simulink library "arc"  (R2023b)
settings: Solver=VariableStepAuto  StartTime=0.0  StopTime=10.0  RelTol=1e-3
values from neighbouring files (symbols this model uses):
  AF = 0.90    (= 0.9)    [FC_scenario_inputData.m]    (also in inputData.m = 70)
  eta2 = 0.95    [FC_scenario_inputData.m]    (also in inputData.m)
  f51 = 0.33    [FC_scenario_inputData.m]    (also in inputData.m)
  f53 = 0.33    [FC_scenario_inputData.m]    (also in inputData.m)
  f54 = 1 - f51 - f53 - f56    (= 0.3399)    [FC_scenario_inputData.m]    (also in inputData.m)
  f56 = 1e-4    (= 0.0001)    [FC_scenario_inputData.m]    (also in inputData.m)
  f96 = 0.1    [FC_scenario_inputData.m]    (also in inputData.m)
  f_dir = 0.7    [FC_scenario_inputData.m]    (also in inputData.m = 0.3)
  f_permanent_trap = f_permanent_trap_array(i)    [parametric_analysis_trapping.m]
  fp3 = 1e-4    (= 0.0001)    [FC_scenario_inputData.m]    (also in inputData.m; parametric_analysis_f_p_trap.m = f_p(i))
  fp4 = 1e-4    (= 0.0001)    [FC_scenario_inputData.m]    (also in inputData.m; parametric_analysis_f_p_trap.m = f_p(i))
  I_s_0 = 1.85    [fuelCycleSimulator.m]    (also in parametric_analysis_f_p_trap.m = 0.8; utilities.m = I_s_0 - abs(margin) + inventory_accuracy)
  lambda = 1.73e-9    (= 1.73e-09)    [FC_scenario_inputData.m]    (also in inputData.m)
  M_structural = V_structural * rho_structural/1e3    (= 21350)    [inputData_trapping.m]
  M_tungsten = V_tungsten * rho_tungsten/1e3    (= 6755)    [inputData_trapping.m]
  m_u = 1.6e-27    [inputData_trapping.m]
  N_dot = 9.3e-7    (= 9.3e-07)    [FC_scenario_inputData.m]    (also in inputData.m)
  n_solute_tungsten = 6    [inputData_trapping.m]
  n_structural = (rho_structural*1e6) / PM_structural * N_a    (= 7.36894684052e+28)    [inputData_trapping.m]
  n_trap = n_trap_array(j)    [parametric_analysis_trapping.m]
  n_trap_structural = n_trap_vcrti    (= 0.0001)    [inputData_trapping.m]    (also in parametric_analysis_trapping.m = n_trap_array(j))
  n_tungsten = (rho_tungsten*1e6) / PM_tungsten * N_a    (= 6.32342763874e+28)    [inputData_trapping.m]
  PM_structural = PM_vcrti    (= 49.85)    [inputData_trapping.m]
  PM_tritium = 3    [inputData_trapping.m]
  PM_tungsten = 183.8    [inputData_trapping.m]
  T1 = 1/((1 + epsi)/tau1 + lambda)    [FC_scenario_inputData.m]    (also in inputData.m)
  T12 = 1/((1 + epsi)/tau12 + lambda)    [FC_scenario_inputData.m]    (also in inputData.m)
  T2 = 1/((1 + epsi)/tau2 + lambda)    [FC_scenario_inputData.m]    (also in inputData.m)
  T3 = 1/((1 + 0)/tau3 + lambda)    [FC_scenario_inputData.m]    (also in inputData.m)
  T4 = 1/((1 + 0)/tau4 + lambda)    [FC_scenario_inputData.m]    (also in inputData.m)
  T5 = 1/((1 + epsi)/tau5 + lambda)    [FC_scenario_inputData.m]    (also in inputData.m)
  T6 = 1/((1 + epsi)/tau6 + lambda)    [FC_scenario_inputData.m]    (also in inputData.m)
  T7 = 1/((1 + epsi)/tau7 + lambda)    [FC_scenario_inputData.m]    (also in inputData.m)
  T9 = 1/((1 + epsi)/tau9 + lambda)    [FC_scenario_inputData.m]    (also in inputData.m)
  T_replacement = 1.7*8760*3600    (= 53611200)    [inputData.m]
  tau1 = 1.25*3600    (= 4500)    [FC_scenario_inputData.m]    (also in inputData.m)
  tau12 = 100    [FC_scenario_inputData.m]    (also in inputData.m)
  tau2 = 1*24*3600    (= 86400)    [FC_scenario_inputData.m]    (also in inputData.m)
  tau3 = 1000    [FC_scenario_inputData.m]    (also in inputData.m)
  tau4 = 1000    [FC_scenario_inputData.m]    (also in inputData.m)
  tau5 = 1000    [FC_scenario_inputData.m]    (also in inputData.m)
  tau6 = 3600    [FC_scenario_inputData.m]    (also in inputData.m)
  tau7 = 600    [FC_scenario_inputData.m]    (also in inputData.m)
  tau8 = 0.1*3600    (= 360)    [FC_scenario_inputData.m]    (also in inputData.m = 3600)
  tau9 = 0.9*3600    (= 3240)    [FC_scenario_inputData.m]    (also in inputData.m = 10800)
  tau_detrap_structural = 1 / nu_detrap_structural* relaxation_coefficient    [inputData_trapping.m]
  tau_detrap_tungsten = 1 ./ nu_detrap* relaxation_coefficient    [inputData_trapping.m]
  tau_trap_structural = 1/nu_trap_structural * relaxation_coefficient    [inputData_trapping.m]
  tau_trap_tungsten = 1/nu_trap * relaxation_coefficient    [inputData_trapping.m]
  TBE = 0.02    [FC_scenario_inputData.m]    (also in inputData.m; parametric_analysis_f_p_trap.m = TBE_array(j); parametric_analysis_trapping.m)
  TBR = 1.096    [fuelCycleSimulator.m]    (also in parametric_analysis_f_p_trap.m = 1.048; parametric_analysis_trapping.m = 1.06; utilities.m = TBR_start)
  V_structural = 3.5e6    (= 3500000)    [inputData_trapping.m]
undefined symbols (not defined in the file or in its folder): f_permanent_trap_structural, n_solute, tau_detrap, tau_permanent, tau_permanent_structural
libraries: $bdroot x4
settings Model: Creator=smesc  LastModifiedBy=meschini
settings OptimizationCC: ReuseModelBlockBuffer=off
settings ModelReferenceCC: EnableRefExpFcnMdlSchedulingChecks=on

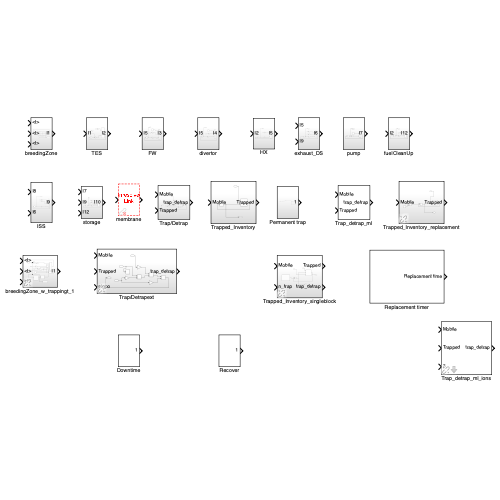
[thumbnail: Simulink's stored preview of the top-level diagram]
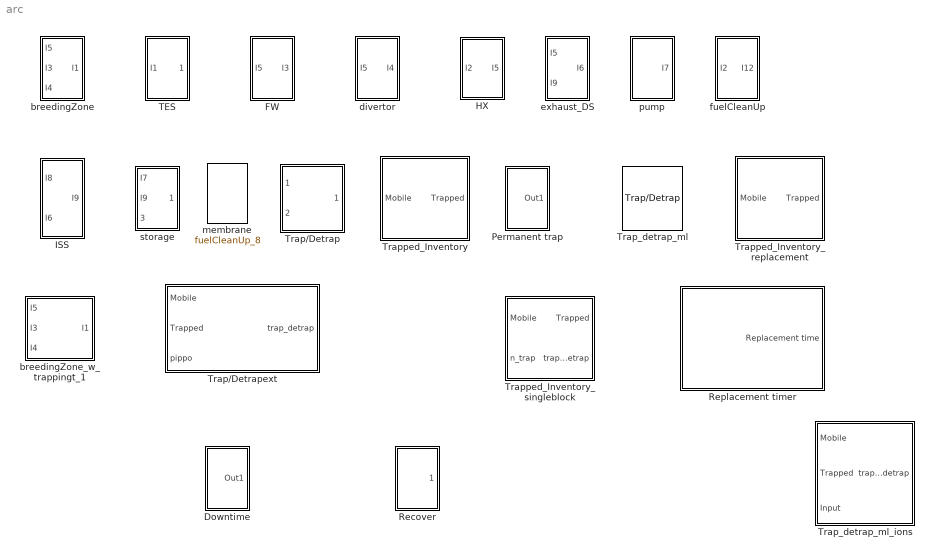
== system arc ==
  Downtime : Subsystem  mask{T_shutdown=0, T_restart=0}
      mask prompts: T_shutdown "Time at which reactor is shutdown"; T_restart "Time at which reactor restarts"
  FW : Subsystem
      settings: LibrarySourceBlock=arc/FW_3
  HX : Subsystem
  ISS : Subsystem
      settings: LibrarySourceBlock=arc/ISS_9
  Permanent trap : Subsystem
  Recover : Subsystem  mask{T_recover_start=0, T_recover_stop=0}
      mask prompts: T_recover_start "Start recover phase"; T_recover_stop "Stop recover phase"
  Replacement timer : Subsystem  mask{T_replacement=T_replacement}
      mask prompts: T_replacement "Replacement time"
  TES : Subsystem
      settings: LibrarySourceBlock=arc/TES_2
  Trap/Detrap : Subsystem
  Trap/Detrapext : Subsystem  AncestorBlock=arc/Trap//Detrap
  Trap_detrap_ml : $bdroot/Trap//Detrap  mask{n_trap=0, tau_trap=0, tau_detrap=0, n_solute=0, PM_host=0, PM_tritium=0, M_host=0}
      mask prompts: n_trap "Trap density"; tau_trap "Tau trap"; tau_detrap "Tau detrap"; PM_host "PM host"; PM_tritium "PM T"
  Trap_detrap_ml_ions : Subsystem  AncestorBlock=arc/Trapped_Inventory_singleblock/Trap_detrap_ml2  mask{tau_trap=tau_trap_tungsten, tau_detrap=tau_detrap_tungsten(1), n_solute=n_solute_tungsten, PM_host=PM_tungsten, PM_tritium=PM_tritium, M_host=M_tungsten, fp=0}
      mask prompts: tau_trap "Tau trap"; tau_detrap "Tau detrap"; PM_host "PM host"; PM_tritium "PM T"; fp "Ions impinging to walls"
  Trapped_Inventory : Subsystem
  Trapped_Inventory_replacement : Subsystem  AncestorBlock=arc/Trapped_Inventory
  Trapped_Inventory_singleblock : Subsystem  AncestorBlock=arc/Trapped_Inventory
  breedingZone : Subsystem
      settings: LibrarySourceBlock=arc/breedingZone_1
  breedingZone_w_trappingt_1 : Subsystem  AncestorBlock=arc/breedingZone_1
      settings: LibrarySourceBlock=arc/breedingZone_1
  divertor : Subsystem
      settings: LibrarySourceBlock=arc/divertor_4
  exhaust_DS : Subsystem
  fuelCleanUp : Subsystem
      settings: LibrarySourceBlock=arc/fuelCleanUp_8
  membrane : $bdroot/fuelCleanUp_8  SystemSampleTime=-1  SSRTWFcnClass=[]  VariantActivationTime=update diagram  Latency=0  AutoFrameSizeCalculation=off
      settings: LibrarySourceBlock=arc/fuelCleanUp_8
  pump : Subsystem
      settings: LibrarySourceBlock=arc/pump_7
  storage : Subsystem
      settings: LibrarySourceBlock=arc/storage_10

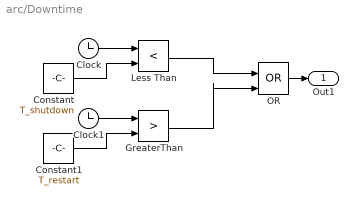
== system arc/Downtime ==
  Clock : Clock
  Clock1 : Clock
  Constant : Constant  Value=T_shutdown
  Constant1 : Constant  Value=T_restart
  GreaterThan : RelationalOperator  Operator=>  OutDataTypeStr=boolean  RndMeth=Simplest  InputSameDT=off
  Less Than : RelationalOperator  Operator=<  OutDataTypeStr=boolean  RndMeth=Simplest  InputSameDT=off
  OR : Logic  Operator=OR  IconShape=distinctive  AllPortsSameDT=off  OutDataTypeStr=boolean
  Out1 : Outport
  wires:
  OR/1 -> Out1/1
  Constant/1 -> Less Than/2
  GreaterThan/1 -> OR/2
  Clock/1 -> Less Than/1
  Clock1/1 -> GreaterThan/1
  Constant1/1 -> GreaterThan/2
  Less Than/1 -> OR/1

== system arc/FW ==
  I5 : Inport
  Add : Sum  Inputs=++-
  Gain : Gain  Gain=f53/tau5
  Gain2 : Gain  Gain=1/T3
  Integrator : Integrator
  Pulse Generator : DiscretePulseGenerator  PulseType=Time based  Amplitude=fp3*N_dot/TBE  Period=1800  PulseWidth=AF
  I3 : Outport
  wires:
  I5/1 -> Gain/1
  Gain/1 -> Add/2
  Add/1 -> Integrator/1  "I_dot"
  Integrator/1 -> Gain2/1, I3/1  "I"
  Pulse Generator/1 -> Add/1
  Gain2/1 -> Add/3

== system arc/HX ==
  I2 : Inport
  Add : Sum  Inputs=+-
  Gain : Gain  Gain=(1-eta2)/tau2
  Gain3 : Gain  Gain=1/T5
  Integrator : Integrator
  I5 : Outport
  wires:
  I2/1 -> Gain/1
  Gain3/1 -> Add/2
  Gain/1 -> Add/1
  Add/1 -> Integrator/1  "I_dot"
  Integrator/1 -> I5/1, Gain3/1  "I"

== system arc/ISS ==
  I8 : Inport
  I6 : Inport  Port=2
  Add : Sum  Inputs=++-
  Gain : Gain  Gain=1/tau8
  Gain1 : Gain  Gain=1/tau6
  Gain4 : Gain  Gain=1/T9
  Integrator : Integrator
  I9 : Outport
  wires:
  Gain4/1 -> Add/3
  Gain/1 -> Add/1
  Integrator/1 -> I9/1, Gain4/1  "I"
  Add/1 -> Integrator/1  "I_dot"
  I6/1 -> Gain1/1
  Gain1/1 -> Add/2
  I8/1 -> Gain/1

== system arc/Permanent trap ==
  Clock : Clock
  Exp : Math
  Gain1 : Gain  Gain=-1/tau_permanent
  Gain3 : Gain  Gain=f_permanent_trap*n_trap*n_tungsten*3*m_u*1/tau_permanent
  Scope : Scope
  Out1 : Outport
  wires:
  Exp/1 -> Gain3/1
  Gain3/1 -> Scope/1, Out1/1
  Clock/1 -> Gain1/1
  Gain1/1 -> Exp/1

== system arc/Recover ==
  AND : Logic  IconShape=distinctive  AllPortsSameDT=off  OutDataTypeStr=boolean
  Clock : Clock
  Clock1 : Clock
  Constant : Constant  Value=T_recover_stop
  Constant1 : Constant  Value=T_recover_start
  GreaterThan : RelationalOperator  Operator=>  OutDataTypeStr=boolean  RndMeth=Simplest  InputSameDT=off
  Less Than : RelationalOperator  Operator=<  OutDataTypeStr=boolean  RndMeth=Simplest  InputSameDT=off
  Output : Outport
  wires:
  GreaterThan/1 -> AND/2
  Clock/1 -> Less Than/1
  AND/1 -> Output/1
  Clock1/1 -> GreaterThan/1
  Constant/1 -> Less Than/2
  Constant1/1 -> GreaterThan/2
  Less Than/1 -> AND/1

== system arc/Replacement timer ==
  Clock : Clock
  Constant1 : Constant  Value=T_replacement
  Rem : Math  Operator=mod
  Replacement time : Outport
  wires:
  Clock/1 -> Rem/1
  Constant1/1 -> Rem/2
  Rem/1 -> Replacement time/1

== system arc/TES ==
  I1 : Inport
  Add : Sum  Inputs=+-
  Gain : Gain  Gain=1/T2
  Gain1 : Gain  Gain=1/tau1
  Integrator : Integrator
  Output : Outport
  wires:
  Add/1 -> Integrator/1  "I_dot"
  Integrator/1 -> Output/1, Gain/1  "I2"
  Gain1/1 -> Add/1
  I1/1 -> Gain1/1
  Gain/1 -> Add/2

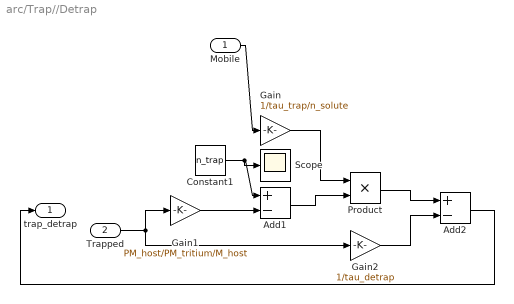
== system arc/Trap//Detrap ==
  Mobile : Inport
  Trapped : Inport  Port=2
  Add1 : Sum  Inputs=+-
  Add2 : Sum  Inputs=+-
  Constant1 : Constant  Value=n_trap
  Gain : Gain  Gain=1/tau_trap/n_solute
  Gain1 : Gain  Gain=PM_host/PM_tritium/M_host
  Gain2 : Gain  Gain=1/tau_detrap
  Product : Product
  Scope : Scope
  trap_detrap : Outport
  wires:
  Product/1 -> Add2/1
  Add2/1 -> trap_detrap/1
  Mobile/1 -> Gain/1
  Gain/1 -> Product/1
  Constant1/1 -> Scope/1, Add1/1
  Gain2/1 -> Add2/2
  Add1/1 -> Product/2
  Gain1/1 -> Add1/2
  Trapped/1 -> Gain2/1, Gain1/1

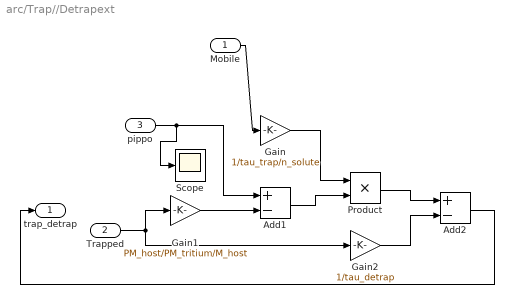
== system arc/Trap//Detrapext ==
  Mobile : Inport
  Trapped : Inport  Port=2
  pippo : Inport  Port=3
  Add1 : Sum  Inputs=+-
  Add2 : Sum  Inputs=+-
  Gain : Gain  Gain=1/tau_trap/n_solute
  Gain1 : Gain  Gain=PM_host/PM_tritium/M_host
  Gain2 : Gain  Gain=1/tau_detrap
  Product : Product
  Scope : Scope
  trap_detrap : Outport
  wires:
  Product/1 -> Add2/1
  Add2/1 -> trap_detrap/1
  Mobile/1 -> Gain/1
  Gain/1 -> Product/1
  pippo/1 -> Scope/1, Add1/1
  Gain2/1 -> Add2/2
  Add1/1 -> Product/2
  Gain1/1 -> Add1/2
  Trapped/1 -> Gain2/1, Gain1/1

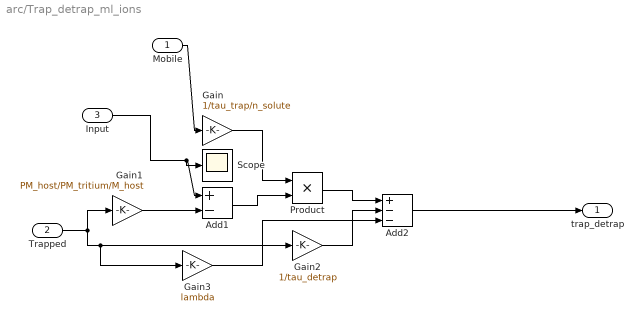
== system arc/Trap_detrap_ml_ions ==
  Mobile : Inport
  Trapped : Inport  Port=2
  Input : Inport  Port=3
  Add1 : Sum  Inputs=+-
  Add2 : Sum  Inputs=+--
  Gain : Gain  Gain=1/tau_trap/n_solute
  Gain1 : Gain  Gain=PM_host/PM_tritium/M_host
  Gain2 : Gain  Gain=1/tau_detrap
  Gain3 : Gain  Gain=lambda
  Product : Product
  Scope : Scope
  trap_detrap : Outport
  wires:
  Trapped/1 -> Gain1/1, Gain2/1, Gain3/1
  Gain1/1 -> Add1/2
  Add1/1 -> Product/2
  Input/1 -> Add1/1, Scope/1
  Gain/1 -> Product/1
  Mobile/1 -> Gain/1
  Add2/1 -> trap_detrap/1
  Product/1 -> Add2/1
  Gain2/1 -> Add2/2
  Gain3/1 -> Add2/3

== system arc/Trapped_Inventory ==
  Mobile : Inport
  Integrator1 : Integrator
  Trap/Detrap : Subsystem
  Trapped : Outport
  wires:
  Integrator1/1 -> Trapped/1, Trap/Detrap/2(In2)
  Mobile/1 -> Trap/Detrap/1(In1)
  Trap/Detrap/1(Out1) -> Integrator1/1

== system arc/Trapped_Inventory_replacement ==
  Mobile : Inport
  Clock : Clock
  Constant1 : Constant  Value=T_replacement
  Integrator1 : Integrator  ExternalReset=falling
  Rem : Math  Operator=mod
  Trap_detrap_ml : $bdroot/Trap_detrap_ml  n_trap=n_trap_structural  tau_trap=tau_trap_structural  tau_detrap=tau_detrap_structural  n_solute=n_solute  PM_host=PM_structural  PM_tritium=PM_tritium  M_host=M_structural
  Trapped : Outport
  wires:
  Mobile/1 -> Trap_detrap_ml/1
  Integrator1/1 -> Trap_detrap_ml/2, Trapped/1
  Clock/1 -> Rem/1
  Rem/1 -> Integrator1/2
  Constant1/1 -> Rem/2
  Trap_detrap_ml/1 -> Integrator1/1

== system arc/Trapped_Inventory_singleblock ==
  Mobile : Inport
  n_trap : Inport  Port=2
  Integrator1 : Integrator  ExternalReset=falling
  Replacement timer : $bdroot/Replacement timer  T_replacement=T_replacement
  Trap_detrap_ml2 : Subsystem  AncestorBlock=arc/Trap_detrap_ml  mask{tau_trap=tau_trap_structural, tau_detrap=tau_detrap_tungsten(3), n_solute=n_solute, PM_host=PM_structural, PM_tritium=PM_tritium, M_host=M_structural}
      mask prompts: tau_trap "Tau trap"; tau_detrap "Tau detrap"; PM_host "PM host"; PM_tritium "PM T"
  Trapped : Outport
  trap_detrap : Outport  Port=2
  wires:
  Integrator1/1 -> Trap_detrap_ml2/2(Trapped), Trapped/1
  Mobile/1 -> Trap_detrap_ml2/1(Mobile)
  Trap_detrap_ml2/1(trap_detrap) -> trap_detrap/1, Integrator1/1
  n_trap/1 -> Trap_detrap_ml2/3(Input)
  Replacement timer/1 -> Integrator1/2

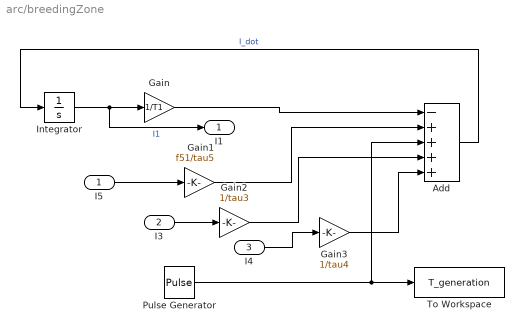
== system arc/breedingZone ==
  I5 : Inport
  I3 : Inport  Port=2
  I4 : Inport  Port=3
  Add : Sum  Inputs=-++++
  Gain : Gain  Gain=1/T1
  Gain1 : Gain  Gain=f51/tau5
  Gain2 : Gain  Gain=1/tau3
  Gain3 : Gain  Gain=1/tau4
  Integrator : Integrator
  Pulse Generator : DiscretePulseGenerator  PulseType=Time based  Amplitude=N_dot * TBR  Period=1800  PulseWidth=AF
  To Workspace : ToWorkspace  VariableName=T_generation  SaveFormat=Timeseries  SampleTime=-1
  I1 : Outport
  wires:
  Gain3/1 -> Add/5
  I4/1 -> Gain3/1
  Gain2/1 -> Add/4
  I3/1 -> Gain2/1
  Pulse Generator/1 -> To Workspace/1, Add/3
  I5/1 -> Gain1/1
  Gain/1 -> Add/1
  Integrator/1 -> I1/1, Gain/1  "I1"
  Gain1/1 -> Add/2
  Add/1 -> Integrator/1  "I_dot"

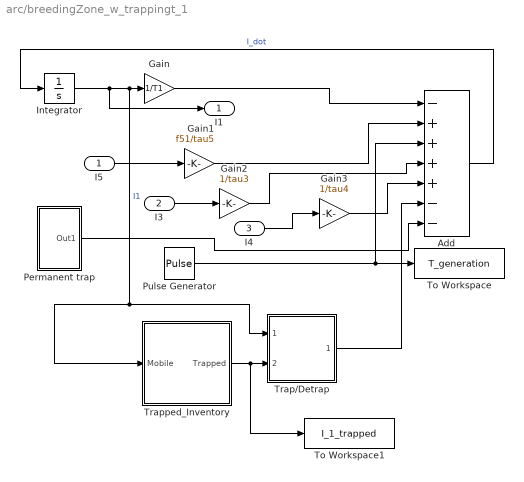
== system arc/breedingZone_w_trappingt_1 ==
  I5 : Inport
  I3 : Inport  Port=2
  I4 : Inport  Port=3
  Add : Sum  Inputs=-++++--
  Gain : Gain  Gain=1/T1
  Gain1 : Gain  Gain=f51/tau5
  Gain2 : Gain  Gain=1/tau3
  Gain3 : Gain  Gain=1/tau4
  Integrator : Integrator
  Permanent trap : Subsystem
  Pulse Generator : DiscretePulseGenerator  PulseType=Time based  Amplitude=N_dot * TBR  Period=1800  PulseWidth=AF
  To Workspace : ToWorkspace  VariableName=T_generation  SaveFormat=Timeseries  SampleTime=-1
  To Workspace1 : ToWorkspace  VariableName=I_1_trapped  SampleTime=-1
  Trap/Detrap : Subsystem  AncestorBlock=arc/Trap//Detrap
  Trapped_Inventory : Subsystem  AncestorBlock=arc/Trapped_Inventory
  I1 : Outport
  wires:
  Add/1 -> Integrator/1  "I_dot"
  Gain1/1 -> Add/2
  Integrator/1 -> Trapped_Inventory/1(Mobile), Trap/Detrap/1(Mobile), Gain/1, I1/1  "I1"
  Gain/1 -> Add/1
  I5/1 -> Gain1/1
  Pulse Generator/1 -> Add/3, To Workspace/1
  I3/1 -> Gain2/1
  Gain2/1 -> Add/4
  I4/1 -> Gain3/1
  Gain3/1 -> Add/5
  Trapped_Inventory/1(Trapped) -> To Workspace1/1, Trap/Detrap/2(Trapped)
  Trap/Detrap/1(trap_detrap) -> Add/6
  Permanent trap/1(Out1) -> Add/7

== system arc/divertor ==
  I5 : Inport
  Add : Sum  Inputs=++-
  Gain : Gain  Gain=f54/tau5
  Gain2 : Gain  Gain=1/T4
  Integrator : Integrator
  Pulse Generator : DiscretePulseGenerator  PulseType=Time based  Amplitude=fp4*N_dot/TBE  Period=1800  PulseWidth=AF
  I4 : Outport
  wires:
  I5/1 -> Gain/1
  Gain2/1 -> Add/3
  Add/1 -> Integrator/1  "I_dot"
  Integrator/1 -> I4/1, Gain2/1  "I"
  Gain/1 -> Add/2
  Pulse Generator/1 -> Add/1

== system arc/exhaust_DS ==
  I5 : Inport
  I9 : Inport  Port=2
  Add : Sum  Inputs=++-
  Gain : Gain  Gain=f56/tau5
  Gain1 : Gain  Gain=f96/tau9
  Gain2 : Gain  Gain=1/T6
  Integrator : Integrator
  I6 : Outport
  wires:
  Gain/1 -> Add/1
  I5/1 -> Gain/1
  Gain1/1 -> Add/2
  Add/1 -> Integrator/1  "I_dot"
  Gain2/1 -> Add/3
  Integrator/1 -> I6/1, Gain2/1  "I"
  I9/1 -> Gain1/1

== system arc/fuelCleanUp ==
  I2 : Inport
  Add : Sum  Inputs=+-
  Gain : Gain  Gain=eta2/tau2
  Gain1 : Gain  Gain=1/T12
  Integrator : Integrator
  I12 : Outport
  wires:
  Gain/1 -> Add/1
  Integrator/1 -> I12/1, Gain1/1  "I"
  Add/1 -> Integrator/1  "I_dot"
  Gain1/1 -> Add/2
  I2/1 -> Gain/1

== system arc/pump ==
  Add : Sum  Inputs=+-
  Gain : Gain  Gain=1/T7
  Integrator : Integrator
  Pulse Generator : DiscretePulseGenerator  PulseType=Time based  Amplitude=(1-TBE-fp3-fp4)*N_dot/TBE  Period=1800  PulseWidth=AF
  I7 : Outport
  wires:
  Add/1 -> Integrator/1  "I_dot"
  Pulse Generator/1 -> Add/1
  Integrator/1 -> I7/1, Gain/1  "I7"
  Gain/1 -> Add/2

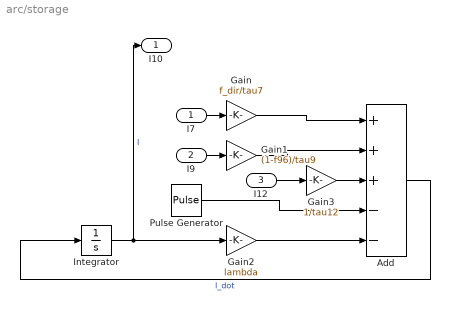
== system arc/storage ==
  I7 : Inport
  I9 : Inport  Port=2
  I12 : Inport  Port=3
  Add : Sum  Inputs=+++--
  Gain : Gain  Gain=f_dir/tau7
  Gain1 : Gain  Gain=(1-f96)/tau9
  Gain2 : Gain  Gain=lambda
  Gain3 : Gain  Gain=1/tau12
  Integrator : Integrator  InitialCondition=I_s_0
  Pulse Generator : DiscretePulseGenerator  PulseType=Time based  Amplitude=N_dot/TBE  Period=1800  PulseWidth=AF
  I10 : Outport
  wires:
  Gain3/1 -> Add/3
  I12/1 -> Gain3/1
  Pulse Generator/1 -> Add/4
  Gain/1 -> Add/1
  Gain1/1 -> Add/2
  I7/1 -> Gain/1
  Gain2/1 -> Add/5
  Add/1 -> Integrator/1  "I_dot"
  I9/1 -> Gain1/1
  Integrator/1 -> I10/1, Gain2/1  "I"

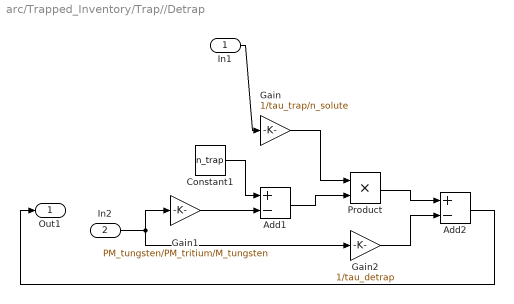
== system arc/Trapped_Inventory/Trap//Detrap ==
  In1 : Inport
  In2 : Inport  Port=2
  Add1 : Sum  Inputs=+-
  Add2 : Sum  Inputs=+-
  Constant1 : Constant  Value=n_trap
  Gain : Gain  Gain=1/tau_trap/n_solute
  Gain1 : Gain  Gain=PM_tungsten/PM_tritium/M_tungsten
  Gain2 : Gain  Gain=1/tau_detrap
  Product : Product
  Out1 : Outport
  wires:
  Product/1 -> Add2/1
  Add2/1 -> Out1/1
  In1/1 -> Gain/1
  Gain/1 -> Product/1
  Constant1/1 -> Add1/1
  Gain2/1 -> Add2/2
  Add1/1 -> Product/2
  Gain1/1 -> Add1/2
  In2/1 -> Gain2/1, Gain1/1

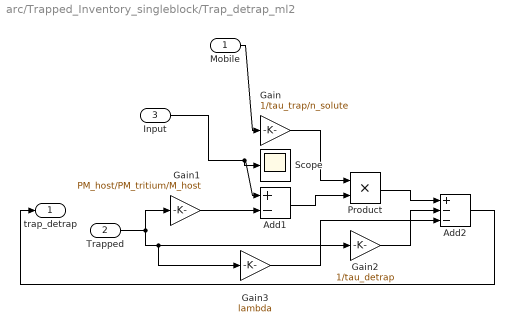
== system arc/Trapped_Inventory_singleblock/Trap_detrap_ml2 ==
  Mobile : Inport
  Trapped : Inport  Port=2
  Input : Inport  Port=3
  Add1 : Sum  Inputs=+-
  Add2 : Sum  Inputs=+--
  Gain : Gain  Gain=1/tau_trap/n_solute
  Gain1 : Gain  Gain=PM_host/PM_tritium/M_host
  Gain2 : Gain  Gain=1/tau_detrap
  Gain3 : Gain  Gain=lambda
  Product : Product
  Scope : Scope
  trap_detrap : Outport
  wires:
  Product/1 -> Add2/1
  Add2/1 -> trap_detrap/1
  Mobile/1 -> Gain/1
  Gain/1 -> Product/1
  Input/1 -> Scope/1, Add1/1
  Gain2/1 -> Add2/2
  Add1/1 -> Product/2
  Gain1/1 -> Add1/2
  Trapped/1 -> Gain3/1, Gain2/1, Gain1/1
  Gain3/1 -> Add2/3

== system arc/breedingZone_w_trappingt_1/Permanent trap ==
  Add : Sum  Inputs=+-
  Clock : Clock
  Constant : Constant
  Exp : Math
  Gain1 : Gain  Gain=-1/tau_permanent_structural
  Gain3 : Gain  Gain=f_permanent_trap_structural*n_trap_structural*n_structural*3*m_u*1*(V_structural/2)
  Scope : Scope
  Out1 : Outport
  wires:
  Gain3/1 -> Scope/1, Out1/1
  Clock/1 -> Gain1/1
  Gain1/1 -> Exp/1
  Add/1 -> Gain3/1
  Constant/1 -> Add/1
  Exp/1 -> Add/2

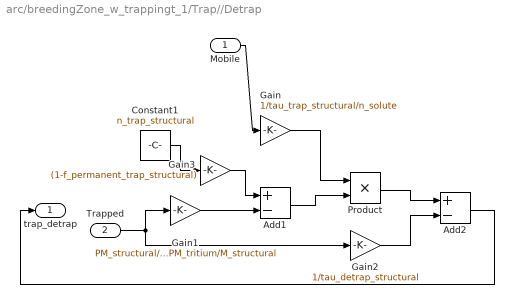
== system arc/breedingZone_w_trappingt_1/Trap//Detrap ==
  Mobile : Inport
  Trapped : Inport  Port=2
  Add1 : Sum  Inputs=+-
  Add2 : Sum  Inputs=+-
  Constant1 : Constant  Value=n_trap_structural
  Gain : Gain  Gain=1/tau_trap_structural/n_solute
  Gain1 : Gain  Gain=PM_structural/PM_tritium/M_structural
  Gain2 : Gain  Gain=1/tau_detrap_structural
  Gain3 : Gain  Gain=(1-f_permanent_trap_structural)
  Product : Product
  trap_detrap : Outport
  wires:
  Trapped/1 -> Gain1/1, Gain2/1
  Gain1/1 -> Add1/2
  Add1/1 -> Product/2
  Gain2/1 -> Add2/2
  Gain/1 -> Product/1
  Mobile/1 -> Gain/1
  Add2/1 -> trap_detrap/1
  Product/1 -> Add2/1
  Constant1/1 -> Gain3/1
  Gain3/1 -> Add1/1

== system arc/breedingZone_w_trappingt_1/Trapped_Inventory ==
  Mobile : Inport
  Integrator1 : Integrator
  Trap/Detrap : Subsystem
  Trapped : Outport
  wires:
  Trap/Detrap/1(Out1) -> Integrator1/1
  Mobile/1 -> Trap/Detrap/1(In1)
  Integrator1/1 -> Trap/Detrap/2(In2), Trapped/1

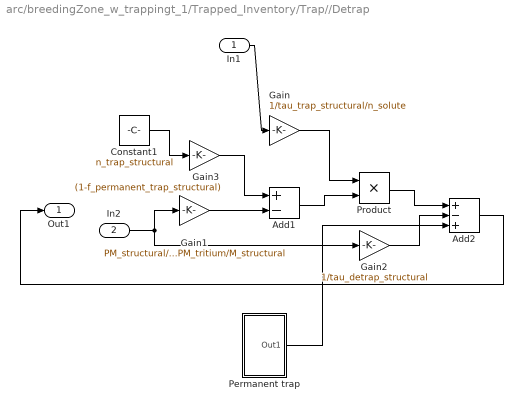
== system arc/breedingZone_w_trappingt_1/Trapped_Inventory/Trap//Detrap ==
  In1 : Inport
  In2 : Inport  Port=2
  Add1 : Sum  Inputs=+-
  Add2 : Sum  Inputs=+-+
  Constant1 : Constant  Value=n_trap_structural
  Gain : Gain  Gain=1/tau_trap_structural/n_solute
  Gain1 : Gain  Gain=PM_structural/PM_tritium/M_structural
  Gain2 : Gain  Gain=1/tau_detrap_structural
  Gain3 : Gain  Gain=(1-f_permanent_trap_structural)
  Permanent trap : Subsystem
  Product : Product
  Out1 : Outport
  wires:
  In2/1 -> Gain1/1, Gain2/1
  Gain1/1 -> Add1/2
  Add1/1 -> Product/2
  Gain2/1 -> Add2/2
  Gain/1 -> Product/1
  In1/1 -> Gain/1
  Add2/1 -> Out1/1
  Product/1 -> Add2/1
  Permanent trap/1(Out1) -> Add2/3
  Constant1/1 -> Gain3/1
  Gain3/1 -> Add1/1

== system arc/breedingZone_w_trappingt_1/Trapped_Inventory/Trap//Detrap/Permanent trap ==
  Add : Sum  Inputs=+-
  Clock : Clock
  Constant : Constant
  Exp : Math
  Gain1 : Gain  Gain=-1/tau_permanent_structural
  Gain3 : Gain  Gain=f_permanent_trap_structural*n_trap_structural*n_structural*3*m_u*1*(V_structural/2)
  Scope : Scope
  Out1 : Outport
  wires:
  Gain3/1 -> Scope/1, Out1/1
  Clock/1 -> Gain1/1
  Gain1/1 -> Exp/1
  Add/1 -> Gain3/1
  Constant/1 -> Add/1
  Exp/1 -> Add/2
